simulink model "p2simulinkLINEAL"  (Simulink 9.1)
settings: Solver=VariableStepAuto  StartTime=0.0  StopTime=10.0  RelTol=1e-3
values from neighbouring files (symbols this model uses):
  b = 0.5    [Problema2.m]    (also in Problema2TF.m)
  Fmeq = k*(ieq^2)/yeq    (= 1.96001568013)    [Problema2.m]    (also in Problema2TF.m)
  g = 9.8    [Problema2.m]    (also in Problema2TF.m)
  ieq = 0.5    [Problema2.m]    (also in Problema2TF.m)
  ki = (2*k*ieq)/yeq    (= 7.8400627205)    [Problema2.m]    (also in Problema2TF.m)
  ky = -k*(ieq^2)/(yeq^2)    (= -7.68332293268)    [Problema2.m]    (also in Problema2TF.m)
  L = 0.01    [Problema2.m]    (also in Problema2TF.m)
  m = 0.2    [Problema2.m]    (also in Problema2TF.m; criterioRouth.m = 4)
  R = 20    [Problema2.m]    (also in Problema2TF.m)
  yeq = 0.2551    [Problema2.m]    (also in Problema2TF.m)
settings Model: Creator=valen  LastModifiedBy=valen
settings DataIOCC: SaveFormat=Dataset
settings OptimizationCC: LifeSpan=auto
settings DebuggingCC: UnderspecifiedInitializationDetection=Simplified  MergeDetectMultiDrivingBlocksExec=error  SFUnexpectedBacktrackingDiag=error  SFNoUnconditionalDefaultTransitionDiag=error  SFExecutionAtInitializationDiag=warning
settings HardwareCC: ProdBitPerPointer=64  ProdBitPerSizeT=64  ProdBitPerPtrDiffT=64  ProdLargestAtomicFloat=Float  ProdIntDivRoundTo=Zero  ProdEndianess=LittleEndian  ProdWordSize=64  ProdHWDeviceType=Intel->x86-64 (Windows64)
settings ModelReferenceCC: PropagateSignalLabelsOutOfModel=on
settings CodeAppCC: StateflowObjectComments=off
settings GRTTargetCC: TargetLangStandard=C99 (ISO)  CombineOutputUpdateFcns=on  GRTInterface=off
settings ConfigComp: CovMetricSettings=dwe  CovHtmlReporting=off  CovSaveCumulativeToWorkspaceVar=off  CovSaveSingleToWorkspaceVar=off  CovExternalEMLEnable=on

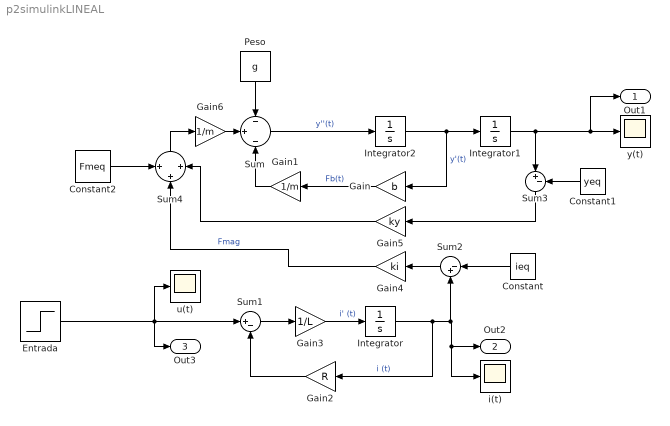
== system p2simulinkLINEAL ==
  Constant : Constant  Value=ieq
  Constant1 : Constant  Value=yeq
  Constant2 : Constant  Value=Fmeq
  Entrada : Step  Time=0  Before=12  After=12  SampleTime=0
  Gain : Gain  Gain=b
  Gain1 : Gain  Gain=1/m
  Gain2 : Gain  Gain=R
  Gain3 : Gain  Gain=1/L
  Gain4 : Gain  Gain=ki
  Gain5 : Gain  Gain=ky
  Gain6 : Gain  Gain=1/m
  Integrator : Integrator
  Integrator1 : Integrator
  Integrator2 : Integrator
  Peso : Constant  Value=g
  Sum : Sum  Inputs=-|+|-
  Sum1 : Sum  Inputs=|+-
  Sum2 : Sum  Inputs=|-+
  Sum3 : Sum  Inputs=|+-
  Sum4 : Sum  Inputs=+|+|+
  i(t) : Scope
  u(t) : Scope
  y(t) : Scope
  Out1 : Outport
  Out2 : Outport  Port=2
  Out3 : Outport  Port=3
  wires:
  Sum/1 -> Integrator2/1  "y''(t)"
  Peso/1 -> Sum/1
  Integrator2/1 -> Integrator1/1, Gain/1  "y'(t)"
  Integrator/1 -> Sum2/2, i(t)/1, Out2/1, Gain2/1  "i (t)"
  Integrator1/1 -> Sum3/1, Out1/1, y(t)/1
  Sum1/1 -> Gain3/1
  Gain2/1 -> Sum1/2
  Gain3/1 -> Integrator/1  "i' (t)"
  Gain/1 -> Gain1/1  "Fb(t)"
  Gain1/1 -> Sum/3
  Constant/1 -> Sum2/1
  Constant1/1 -> Sum3/2
  Sum3/1 -> Gain5/1
  Sum2/1 -> Gain4/1
  Gain5/1 -> Sum4/3
  Gain4/1 -> Sum4/2  "Fmag"
  Constant2/1 -> Sum4/1
  Gain6/1 -> Sum/2
  Sum4/1 -> Gain6/1
  Entrada/1 -> u(t)/1, Out3/1, Sum1/1
